simulink model "model"  (R2023a)
settings: Solver=VariableStepAuto  StartTime=0.0  StopTime=0.01  RelTol=1e-3
settings Model: Creator=Vinay KumarSahu  LastModifiedBy=Vinay KumarSahu

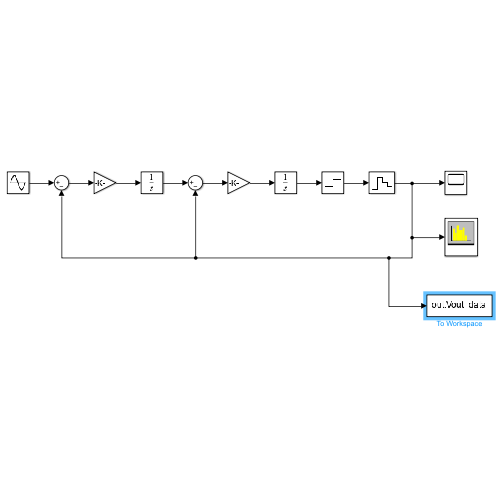
[thumbnail: Simulink's stored preview of the top-level diagram]
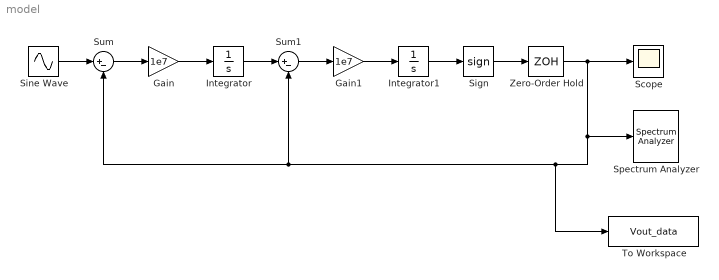
== system model ==
  Gain : Gain  Gain=1e7
  Gain1 : Gain  Gain=1e7
  Integrator : Integrator
  Integrator1 : Integrator
  Scope : Scope
  Sign : Signum
  Sine Wave : Sin  Amplitude=0.5  Frequency=2*pi*1000  SampleTime=0
  Spectrum Analyzer : SpectrumAnalyzer  WindowPosition=[335.000000,142.000000,900.000000,500.000000,]  ScopeFrameLocation=window  PlotAsTwoSidedSpectrum=off  FrequencyScale=Log  YLimits=[-46.74276484,28.27000616]  ColorLimits=[-80 20]  SelectedToolstripTab=spectrumAnalyzerToolstrip.spectrumTab
  Sum : Sum  Inputs=|+-
  Sum1 : Sum  Inputs=|+-
  To Workspace : ToWorkspace  VariableName=Vout_data  SampleTime=-1
  Zero-Order Hold : ZeroOrderHold  SampleTime=1e-7
  wires:
  Sum/1 -> Gain/1
  Integrator/1 -> Sum1/1
  Sum1/1 -> Gain1/1
  Gain1/1 -> Integrator1/1
  Integrator1/1 -> Sign/1
  Sign/1 -> Zero-Order Hold/1
  Sine Wave/1 -> Sum/1
  Zero-Order Hold/1 -> Scope/1, Spectrum Analyzer/1, To Workspace/1, Sum1/2, Sum/2
  Gain/1 -> Integrator/1
